simulink model "openManipulatorBallTracking"  (R2020a)
settings: Solver=VariableStepAuto  StartTime=0.0  StopTime=2  RelTol=1e-3
PreLoadFcn:
  | openManipulatorParameters;
undefined symbols (not defined in the file): position_threshold, TsBall
libraries: OpenManipulatorLib x3
settings Model: Creator=josea  LastModifiedBy=HP
settings DataIOCC: ReturnWorkspaceOutputs=off
settings DebuggingCC: ArithmeticOperatorsInVariantConditions=warning
settings SFSimCC: SimUseLocalCustomCode=off  CustomCodeUndefinedFunction=UseInterfaceOnly
settings RTWCC: RTWUseLocalCustomCode=off
settings SimscapeCC: SimscapeLogType=all  SimscapeLogName=simlog_waypoint_tracking  SimscapeLogLimitData=off
settings ExplorerConfigSet: InternalSimMechanicsExplorerSettings="<ExplorerConfiguration><canonicalview>default</canonicalview><AnimationSetting><BasePlaybackSpeed>1.0</BasePlaybackSpeed><PlaybackSpeedFactor>0.5</PlaybackSpeedFactor></AnimationSetting><TilePanel><TileInfo><Tiles Columns=\"1\" Count=\"1\" Rows=\"1\"><Column Weight=\"1\"/><Row Weight=\"1\"/><Tile Height=\"1\" Width=\"1\" X=\"0\" Y=\"0\"/></Tiles></TileInfo><SceneInfo><SceneViewer><BGColor><R>0.800000011920928955</R><G>0.800000011920928955</G><B>0.800000011920928955</B></BGColor><Camera><DoPerspective>off</DoPerspective><Position><X>0.884423895064342158</X><Y>-0.461753927406516884</Y><Z>0.644809623101804119</Z></Position><Center><X>0.122146713942822532</X><Y>0.0293134737875758097</Y><Z>0.223162487897595768</Z></Center><Up><X>-0.328061437332023642</X><Y>0.268432407534651141</Y><Z>0.905715041235817142</Z></Up><ViewLimDist>1</ViewLimDist><YLim>0.413491851737640914</YLim><XLim>0.495410048780003776</XLim></Camera></SceneViewer></SceneInfo></TilePanel><MechEditorPanel><Cameras/><GfxPanelCameraMap/><VideoCreator><PlaybackSpeedRatio>1.0</PlaybackSpeedRatio><FrameRate>30</FrameRate><VideoFormat>Motion JPEG AVI</VideoFormat><FrameSize>auto</FrameSize></VideoCreator></MechEditorPanel></ExplorerConfiguration>"

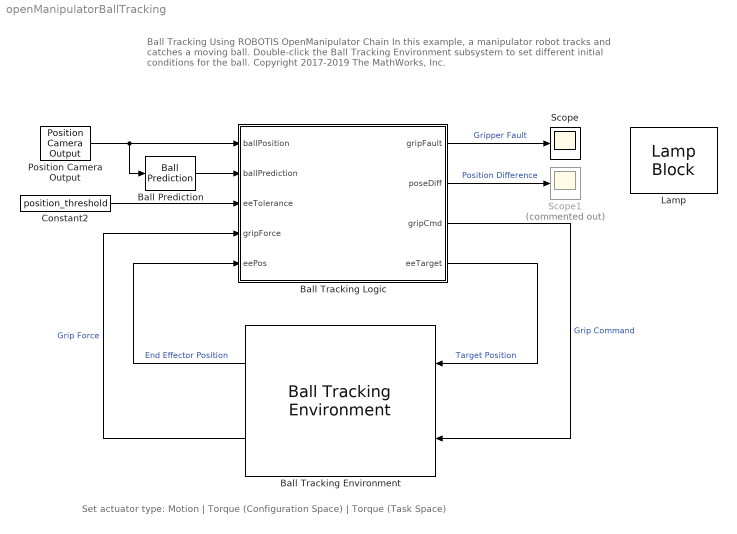
== system openManipulatorBallTracking ==
  note: Ball Tracking Using ROBOTIS OpenManipulator Chain
      |
      | In this example, a manipulator robot tracks and catches a moving ball.
      | Double-click the Ball Tracking Environment subsystem to set different initial conditions for the ball.
      |
      | Copyright 2017-2019 The MathWorks, Inc.
  note: Set actuator type: Motion | Torque (Configuration Space) | Torque (Task Space)
  Ball Prediction : OpenManipulatorLib/Ball Prediction  estDelay=estDelay  time_jump=time_jump  polyOrder=2  Ts=TsBall
  Ball Tracking Environment : OpenManipulatorLib/Ball Tracking Environment  VariantControl=Variant1  BallPositionY=-0.12  BallHeading=34.2  reverse=off  zVel=on
  Ball Tracking Logic : Stateflow chart  TreatAsAtomicUnit=on
  Constant2 : Constant  Value=position_threshold
  Lamp : LampBlock
  Position Camera Output : OpenManipulatorLib/Position Camera Output  SystemSampleTime=-1  Latency=0  AutoFrameSizeCalculation=off
  Scope : Scope
  Scope1 : Scope  Commented=on
  wires:
  Constant2/1 -> Ball Tracking Logic/3(eeTolerance)
  Ball Prediction/1 -> Ball Tracking Logic/2(ballPrediction)
  Ball Tracking Logic/4(eeTarget) -> Ball Tracking Environment/1  "Target Position"
  Ball Tracking Logic/2(poseDiff) -> Scope1/1  "Position Difference"
  Ball Tracking Environment/1 -> Ball Tracking Logic/5(eePos)  "End Effector Position"
  Ball Tracking Logic/1(gripFault) -> Scope/1  "Gripper Fault"
  Position Camera Output/1 -> Ball Tracking Logic/1(ballPosition), Ball Prediction/1
  Ball Tracking Logic/3(gripCmd) -> Ball Tracking Environment/2  "Grip Command"
  Ball Tracking Environment/2 -> Ball Tracking Logic/4(gripForce)  "Grip Force"

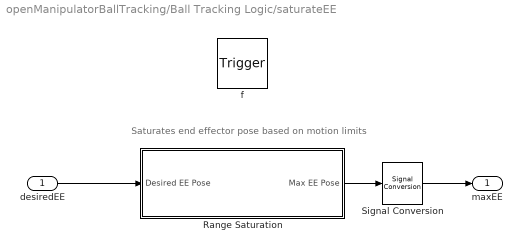
== system openManipulatorBallTracking/Ball Tracking Logic/saturateEE ==
  note: Saturates end effector pose based on motion limits
  desiredEE : Inport  OutDataTypeStr=double  PortDimensions=3
  f : TriggerPort  TriggerType=function-call  VariantControl=(inherit)
      settings: CopyFcn=Stateflow.SLINSF.SimulinkMan.removeBlockPreDeleteFcn  PreDeleteFcn=Stateflow.SLINSF.SimulinkMan.unsafePredeleteFcn
  Range Saturation : Subsystem  mask(End Effector Range Saturation){xUpper=0.3, xLower=0, yUpper=0.22, yLower=-0.22, zUpper=0.25, zLower=0.02}
      mask prompts: xUpper "Max X position"; xLower "Min X position"; yUpper "Max Y position"; yLower "Min Y position"; zUpper "Max Z position"; zLower "Min Z position"
      mask help: This subsystem saturates the end effector position to those within the allowable ranges for the manipulator. This prevents the inverse kinematics algorithms from attempting to find inexistent solution that timeout.
  Signal Conversion : SignalConversion  OverrideOpt=off
  maxEE : Outport  VectorParamsAs1DForOutWhenUnconnected=off
  wires:
  desiredEE/1 -> Range Saturation/1(Desired EE Pose)
  Range Saturation/1(Max EE Pose) -> Signal Conversion/1
  Signal Conversion/1 -> maxEE/1

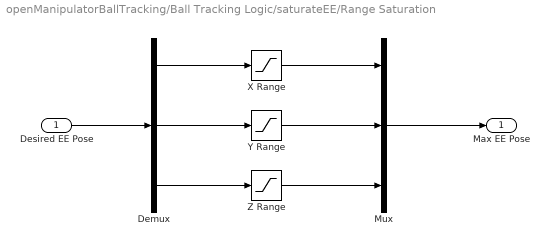
== system openManipulatorBallTracking/Ball Tracking Logic/saturateEE/Range Saturation ==
  Desired EE Pose : Inport
  Demux : Demux  Outputs=3
  Mux : Mux  Inputs=3
  X Range : Saturate  UpperLimit=xUpper  LowerLimit=xLower
  Y Range : Saturate  UpperLimit=yUpper  LowerLimit=yLower
  Z Range : Saturate  UpperLimit=zUpper  LowerLimit=zLower
  Max EE Pose : Outport  VectorParamsAs1DForOutWhenUnconnected=off
  wires:
  Desired EE Pose/1 -> Demux/1
  Demux/2 -> Y Range/1
  Demux/3 -> Z Range/1
  X Range/1 -> Mux/1
  Mux/1 -> Max EE Pose/1
  Z Range/1 -> Mux/3
  Y Range/1 -> Mux/2
  Demux/1 -> X Range/1

== stateflow chart openManipulatorBallTracking/Ball Tracking Logic ==
  settings: updateMethod=DISCRETE  sampleTime=TsBall
  state Gripper [parallel]
    settings: executionOrder=2
    state InTransition
    state CloseGripper
      entry:
      counts=0;
      gripCmd=1;
      during:
      counts=counts+1;
    state OpenGripper
      entry:
      counts=0;
      gripCmd=-1;
      during:
      counts=counts+1;
    state GripperFault
      entry: gripFault=1;
    (default) -> InTransition : {gripFault=0;}
    (junction 101) -> InTransition
    (junction 78) -> InTransition
    (junction 64) -> (junction 101)
    OpenGripper -> (junction 78) [order 1] : [~detectBall(0.5)]
        | {RobotMotion.GripSet}
    (junction 86) -> InTransition
    CloseGripper -> (junction 86) [order 1] : [detectBall(0.5)]
        | {RobotMotion.GripSet}
    InTransition -> (junction 75) : SetGrip
    (junction 75) -> OpenGripper [order 2]
    (junction 75) -> CloseGripper [order 1] : [grabBall]
    CloseGripper -> (junction 96) [order 2] : [counts>=10]
    OpenGripper -> (junction 96) [order 2] : [counts>=10]
    (junction 96) -> GripperFault
    GripperFault -> (junction 64) : {gripCmd=0;}
  state RobotMotion [parallel]
    entry, during:
    poseDiff = abs(eePos-ballPosition);
    settings: executionOrder=1
    state WaitForPrediction
      entry:
      eeTarget = homePose;
      grabBall=0;
    state FollowBall
      entry,during:
      eeTarget=saturateEE(ballPrediction);
    state GrabBall
      entry:
      grabBall=1;
      Gripper.SetGrip
      entry,during:
      eeTarget=saturateEE(ballPrediction);
    state GoHome
      entry,during:
      eeTarget= 0.5*(eeTarget+homePose);
    (default) -> WaitForPrediction
    WaitForPrediction -> FollowBall : [all(ballPrediction ~=0)]
    FollowBall -> WaitForPrediction [order 1] : [any(ballPrediction == 0)]
    FollowBall -> GrabBall [order 2] : [checkBallTolerance && all(ballPrediction ~=0)]
    GrabBall -> GoHome : GripSet
  state maxEE = saturateEE(desiredEE) [function]
  data: reachedBall function_output; isBall function_output; threshold function_input; desiredEE function_input double size=3; maxEE function_output; gripFault output; poseDiff output; ballPosition input size=3; ballPrediction input; eeTolerance input; gripCmd output double size=1; gripForce input; eePos input; counts local; eeTarget output size=3; grabBall local; homePose parameter double size=3
  events: SetGrip local FUNCTION_CALL_EVENT; GripSet local FUNCTION_CALL_EVENT
  function reachedBall = checkBallTolerance:
    | function reachedBall = checkBallTolerance
    | % Checks if the end effector and ball are within a specified position tolerance
    | 
    | if ballPosition(3) < 0.2
    |  reachedBall=abs(eePos(1)-ballPosition(1))<eeTolerance(1) ...
    |     && abs(eePos(2)-ballPosition(2))<eeTolerance(2)...
    |     && abs(eePos(3)-ballPosition(3))<eeTolerance(3);
    | else % Use higher tolerance on Z if ball is airborne
    |      reachedBall=abs(eePos(1)-ballPosition(1))<eeTolerance(1) ...
    |     && abs(eePos(2)-ballPosition(2))<eeTolerance(2)...
    |     && abs(eePos(3)-ballPosition(3))<eeTolerance(3)*4;    
    | end
  function isBall = detectBall(threshold):
    | function isBall = detectBall(threshold)
    | % Checks the presence of a ball based on a minimum force threshold
    | 
    | isBall = all(abs(gripForce)>threshold);
